simulink model "s_alqrd1"  (Simulink 4.00)
settings: Solver=ode5  SolverMode=SingleTasking  StartTime=0.0  StopTime=999999  MaxStep=10  RelTol=1e-3  AbsTol=1e-6
values from neighbouring files (symbols this model uses):
  Ts = 0.5    [abeob1.m]    (also in akalm1.m = 0.25; alqrd1.m = 0.25; kalm2.m; kalm3.m)
  x0 = [5, 0, 0, 0]    [abeob1.m]    (also in alqr1.m; alqrd1.m; apol1.m; estimate_1.m = [1 2 3])
settings Model: LastModifiedBy=Administrator  SaveTime=off  SaveOutput=off  LimitDataPoints=off  BlockReductionOpt=off

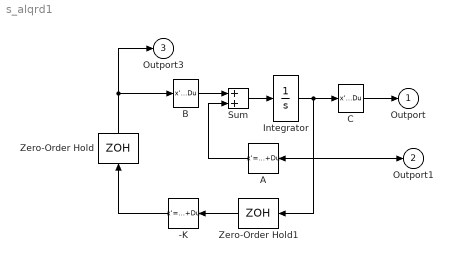
== system s_alqrd1 ==
  -K : StateSpace  Orientation=left  A=[]  B=[]  C=[]  D=K  X0=0  Realization=auto  AbsoluteTolerance=auto  mask(Matrix Gain){@1=-K}
      mask prompts: @1 "Gain matrix:"
      mask help: Matrix Gain.
      mask init:
      | K = @1;
      mask Help: Multiplies input vector by entered matrix to produce output vector (y=Au).
      mask Display: disp('K')
  A : StateSpace  Orientation=left  A=[]  B=[]  C=[]  D=K  X0=0  Realization=auto  AbsoluteTolerance=auto  mask(Matrix Gain){@1=A}
      mask prompts: @1 "Gain matrix:"
      mask help: Matrix Gain.
      mask init:
      | K = @1;
      mask Help: Multiplies input vector by entered matrix to produce output vector (y=Au).
      mask Display: disp('K')
  B : StateSpace  A=[]  B=[]  C=[]  D=K  X0=0  Realization=auto  AbsoluteTolerance=auto  mask(Matrix Gain){@1=B}
      mask prompts: @1 "Gain matrix:"
      mask help: Matrix Gain.
      mask init:
      | K = @1;
      mask Help: Multiplies input vector by entered matrix to produce output vector (y=Au).
      mask Display: disp('K')
  C : StateSpace  A=[]  B=[]  C=[]  D=K  X0=0  Realization=auto  AbsoluteTolerance=auto  mask(Matrix Gain){@1=C}
      mask prompts: @1 "Gain matrix:"
      mask help: Matrix Gain.
      mask init:
      | K = @1;
      mask Help: Multiplies input vector by entered matrix to produce output vector (y=Au).
      mask Display: disp('K')
  Integrator : Integrator  ExternalReset=none  InitialConditionSource=internal  InitialCondition=x0  LimitOutput=off  UpperSaturationLimit=inf  LowerSaturationLimit=-inf  ShowSaturationPort=off  ShowStatePort=off  AbsoluteTolerance=auto
  Sum : Sum  Inputs=++  SaturateOnIntegerOverflow=on
  Zero-Order Hold : ZeroOrderHold  Orientation=up  SampleTime=Ts
  Zero-Order Hold1 : ZeroOrderHold  Orientation=left  SampleTime=Ts
  Outport : Outport  Port=1  InitialOutput=0
  Outport1 : Outport  Port=2  InitialOutput=0
  Outport3 : Outport  Port=3  InitialOutput=0
  wires:
  Zero-Order Hold/1 -> Outport3/1, B/1
  Zero-Order Hold1/1 -> -K/1
  -K/1 -> Zero-Order Hold/1
  C/1 -> Outport/1
  B/1 -> Sum/1
  A/1 -> Sum/2
  Sum/1 -> Integrator/1
  Integrator/1 -> Zero-Order Hold1/1, Outport1/1, A/1, C/1
